simulink model "Quad_model_V1"  (R2021b)
settings: Solver=VariableStepAuto  StartTime=0.0  StopTime=10.0  RelTol=1e-3
values from neighbouring files (symbols this model uses):
  G_1 = [ mot_eff,mot_eff,mot_eff,mot_eff;0,-12.8,0,12.8;2.7,0,-2.7,0;-0.115,0.115,-0.115,0.115]./conv    [Model_Parameters.m]    (also in wls_test.m)
  G_2 = [0,0,0,0;0,0,0,0;0,0,0,0;-0.06,0.06,-0.06,0.06]./conv    [Model_Parameters.m]    (also in wls_test.m)
  H_z_den = [1]    [Model_Parameters.m]
  H_z_num = [1]    [Model_Parameters.m]
  Hz2rads = 6.28    [Model_Parameters.m]    (also in wls_test.m)
  M = 0.1*1/(1-exp(-20*Ts))    [Model_Parameters.m]
  mot_den = [1]    [Model_Parameters.m]
  mot_num = [1]    [Model_Parameters.m]
  pseudo_g12 = pinv(G_1+G_2)    [Model_Parameters.m]    (also in wls_test.m)
  Ts = 1/500    (= 0.002)    [Model_Parameters.m]
libraries: simulink x1, dspsrcs4 x1
settings Model: Creator=tomasodeponti  LastModifiedBy=tomasodeponti

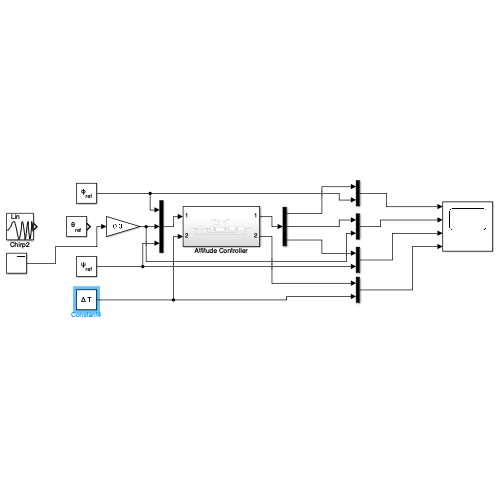
[thumbnail: Simulink's stored preview of the top-level diagram]
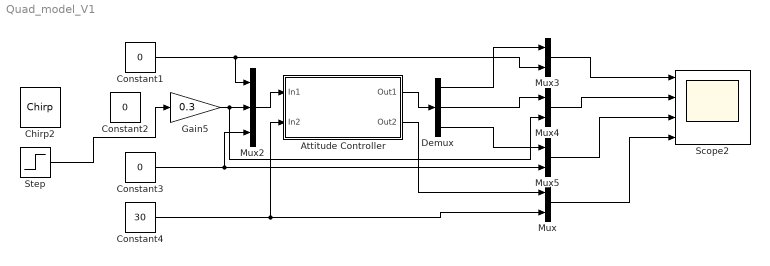
== system Quad_model_V1 ==
  Attitude Controller : Subsystem
  Chirp2 : dspsrcs4/Chirp  sweep=Linear  mode=Unidirectional  f0=0.1  f1=0.5  t1=1  Tsweep=10  phase=0  Ts=Ts  spf=1  datatype=Double  OutputFrames=off
  Constant1 : Constant  Value=0
      mask Display: disp('\phi_{ref}','texmode','on')
  Constant2 : Constant  Value=0
      mask Display: disp('\theta_{ref}','texmode','on')
  Constant3 : Constant  Value=0
      mask Display: disp('\psi_{ref}','texmode','on')
  Constant4 : Constant  Value=30
      mask Display: disp('\Delta T','texmode','on')
  Demux : Demux  Outputs=3
  Gain5 : Gain  Gain=0.3
  Mux{,3..5} (4 alike) : Mux  Inputs=2
  Mux2 : Mux  Inputs=3
  Scope2 : Scope  NumInputPorts=4
  Step : Step  SampleTime=0
  wires:
  Constant1/1 -> Mux2/1, Mux3/2
  Constant3/1 -> Mux2/3, Mux5/2
  Gain5/1 -> Mux4/2, Mux2/2
  Demux/2 -> Mux4/1
  Demux/3 -> Mux5/1
  Mux3/1 -> Scope2/1
  Demux/1 -> Mux3/1
  Mux4/1 -> Scope2/2
  Mux5/1 -> Scope2/3
  Mux2/1 -> Attitude Controller/1(In1)
  Attitude Controller/1(Out1) -> Demux/1
  Step/1 -> Gain5/1
  Constant4/1 -> Attitude Controller/2(In2), Mux/2
  Attitude Controller/2(Out2) -> Mux/1
  Mux/1 -> Scope2/4

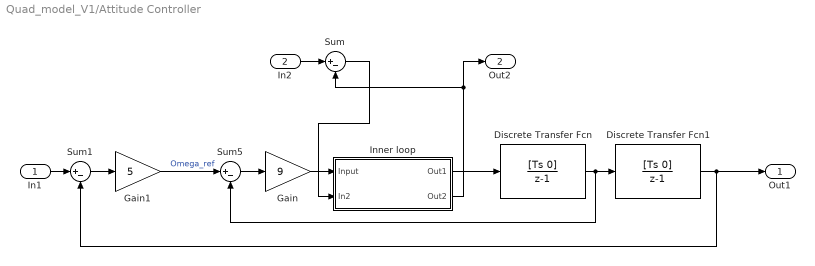
== system Quad_model_V1/Attitude Controller ==
  In1 : Inport
  In2 : Inport  Port=2
  Discrete Transfer Fcn : DiscreteTransferFcn  Numerator=[Ts 0]  Denominator=[1 -1]
  Discrete Transfer Fcn1 : DiscreteTransferFcn  Numerator=[Ts 0]  Denominator=[1 -1]
  Gain : Gain  Gain=9
      mask Display: disp('K_\Omega','texmode','on')
  Gain1 : Gain  Gain=5
      mask Display: disp('K_\eta','texmode','on')
  Inner loop : Subsystem
  Sum : Sum  Inputs=|+-
  Sum1 : Sum  Inputs=|+-
  Sum5 : Sum  Inputs=|+-
  Out1 : Outport
  Out2 : Outport  Port=2
  wires:
  Gain1/1 -> Sum5/1  "Omega_ref"
  Sum5/1 -> Gain/1
  Sum1/1 -> Gain1/1
  Discrete Transfer Fcn/1 -> Sum5/2, Discrete Transfer Fcn1/1
  Gain/1 -> Inner loop/1(Input)
  Inner loop/1(Out1) -> Discrete Transfer Fcn/1
  In1/1 -> Sum1/1
  Discrete Transfer Fcn1/1 -> Out1/1, Sum1/2
  In2/1 -> Sum/1
  Inner loop/2(Out2) -> Sum/2, Out2/1
  Sum/1 -> Inner loop/2(In2)

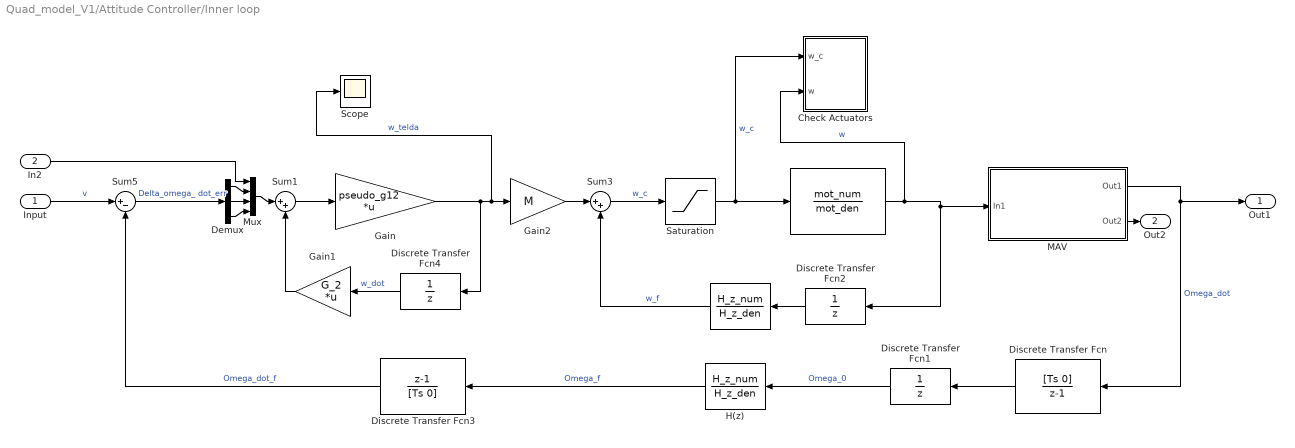
== system Quad_model_V1/Attitude Controller/Inner loop ==
  Input : Inport  PortDimensions=3
  In2 : Inport  Port=2
  " " : DiscreteTransferFcn  Numerator=H_z_num  Denominator=H_z_den  DenCoefDataTypeStr=int16
      mask Display: disp('H(z)')
  "  " : DiscreteTransferFcn  Numerator=mot_num  Denominator=mot_den  DenCoefDataTypeStr=int16
      mask Display: disp('A(z)')
  Check Actuators : Subsystem
  Demux : Demux  Outputs=3
  Discrete Transfer Fcn : DiscreteTransferFcn  Numerator=[Ts 0]  Denominator=[1 -1]
  Discrete Transfer Fcn1 : DiscreteTransferFcn  Denominator=[1 0]
  Discrete Transfer Fcn2 : DiscreteTransferFcn  Denominator=[1 0]
  Discrete Transfer Fcn3 : DiscreteTransferFcn  Numerator=[1 -1]  Denominator=[Ts 0]
  Discrete Transfer Fcn4 : DiscreteTransferFcn  Denominator=[1 0]
  Gain : Gain  Gain=pseudo_g12  Multiplication=Matrix(K*u)
      mask Display: disp('(G1+G2)^+','texmode','on')
  Gain1 : Gain  Gain=G_2  Multiplication=Matrix(K*u)
      mask Display: disp('G2')
  Gain2 : Gain  Gain=M
      mask Display: disp('M')
  H(z) : DiscreteTransferFcn  Numerator=H_z_num  Denominator=H_z_den  DenCoefDataTypeStr=int16
      mask Display: disp('H(z)')
  MAV : Subsystem
      mask Display:
      | %image('C:\Users\Tomaso\Pictures\Screenshots\Screenshot 2021-12-02 165056.png'); % Use "Edit Image" on toolstrip to change.
      | disp('MAV')
  Mux : Mux
  Saturation : Saturate  UpperLimit=150*Hz2rads  LowerLimit=0
  Scope : Scope
  Sum1 : Sum  Inputs=|++
  Sum3 : Sum  Inputs=|++
  Sum5 : Sum  Inputs=|+-
  Out1 : Outport  PortDimensions=3
  Out2 : Outport  Port=2
  wires:
  "  "/1 -> Check Actuators/2(w), Discrete Transfer Fcn2/1, MAV/1(In1)  "w"
  Discrete Transfer Fcn/1 -> Discrete Transfer Fcn1/1
  Discrete Transfer Fcn1/1 -> H(z)/1  "Omega_0"
  Discrete Transfer Fcn2/1 -> " "/1
  Saturation/1 -> Check Actuators/1(w_c), "  "/1  "w_c"
  " "/1 -> Sum3/2  "w_f"
  H(z)/1 -> Discrete Transfer Fcn3/1  "Omega_f"
  Discrete Transfer Fcn3/1 -> Sum5/2  "Omega_dot_f"
  Gain/1 -> Discrete Transfer Fcn4/1, Scope/1, Gain2/1  "w_telda"
  Sum5/1 -> Demux/1  "Delta_omega_ dot_err"
  Sum1/1 -> Gain/1
  Discrete Transfer Fcn4/1 -> Gain1/1  "w_dot"
  Gain1/1 -> Sum1/2
  Input/1 -> Sum5/1  "v"
  Gain2/1 -> Sum3/1
  Sum3/1 -> Saturation/1  "w_c"
  MAV/1(Out1) -> Discrete Transfer Fcn/1, Out1/1  "Omega_dot"
  In2/1 -> Mux/1
  Mux/1 -> Sum1/1
  Demux/1 -> Mux/2
  Demux/2 -> Mux/3
  Demux/3 -> Mux/4
  MAV/2(Out2) -> Out2/1

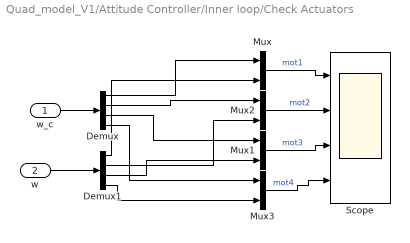
== system Quad_model_V1/Attitude Controller/Inner loop/Check Actuators ==
  w_c : Inport
  w : Inport  Port=2
  Demux : Demux
  Demux1 : Demux
  Mux{,1..3} (4 alike) : Mux  Inputs=2
  Scope : Scope  NumInputPorts=4
  wires:
  Demux1/3 -> Mux1/2
  w_c/1 -> Demux/1
  Demux1/4 -> Mux3/2
  Demux/2 -> Mux2/1
  w/1 -> Demux1/1
  Demux/4 -> Mux3/1
  Mux/1 -> Scope/1  "mot1"
  Demux/3 -> Mux1/1
  Demux1/1 -> Mux/2
  Demux/1 -> Mux/1
  Mux1/1 -> Scope/3  "mot3"
  Demux1/2 -> Mux2/2
  Mux2/1 -> Scope/2  "mot2"
  Mux3/1 -> Scope/4  "mot4"

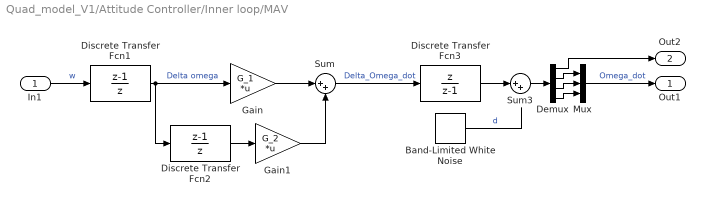
== system Quad_model_V1/Attitude Controller/Inner loop/MAV ==
  In1 : Inport  PortDimensions=4
  Band-Limited White Noise : simulink/Sources/Band-Limited White Noise  Cov=[0.00000001]  Ts=Ts  seed=[23341]
  Demux : Demux
  Discrete Transfer Fcn1 : DiscreteTransferFcn  Numerator=[1 -1]  Denominator=[1 0]
  Discrete Transfer Fcn2 : DiscreteTransferFcn  Numerator=[1 -1]  Denominator=[1 0]
  Discrete Transfer Fcn3 : DiscreteTransferFcn  Numerator=[1 0]  Denominator=[1 -1]
  Gain : Gain  Gain=G_1  Multiplication=Matrix(K*u)
      mask Display: disp('G1')
  Gain1 : Gain  Gain=G_2  Multiplication=Matrix(K*u)
      mask Display: disp('G2')
  Mux : Mux  Inputs=3
  Sum : Sum  Inputs=|++
  Sum3 : Sum  Inputs=|++
  Out1 : Outport  PortDimensions=3
  Out2 : Outport  Port=2
  wires:
  In1/1 -> Discrete Transfer Fcn1/1  "w"
  Discrete Transfer Fcn1/1 -> Discrete Transfer Fcn2/1, Gain/1  "Delta omega"
  Discrete Transfer Fcn2/1 -> Gain1/1
  Gain/1 -> Sum/1
  Gain1/1 -> Sum/2
  Sum/1 -> Discrete Transfer Fcn3/1  "Delta_Omega_dot"
  Discrete Transfer Fcn3/1 -> Sum3/1
  Band-Limited White Noise/1 -> ?  "d"
  Mux/1 -> Out1/1  "Omega_dot"
  Sum3/1 -> Demux/1
  Demux/4 -> Mux/3
  Demux/3 -> Mux/2
  Demux/2 -> Mux/1
  Demux/1 -> Out2/1
